simulink model "drone_nonlinear_full_identification2"  (R2018a)
settings: Solver=VariableStepAuto  StartTime=0.0  StopTime=40  RelTol=1e-3
undefined symbols (not defined in the file): g, Ix, Iy, Iz, m, simulation_sampling_ts
libraries: simulink x4
settings Model: Creator=ros  LastModifiedBy=ros

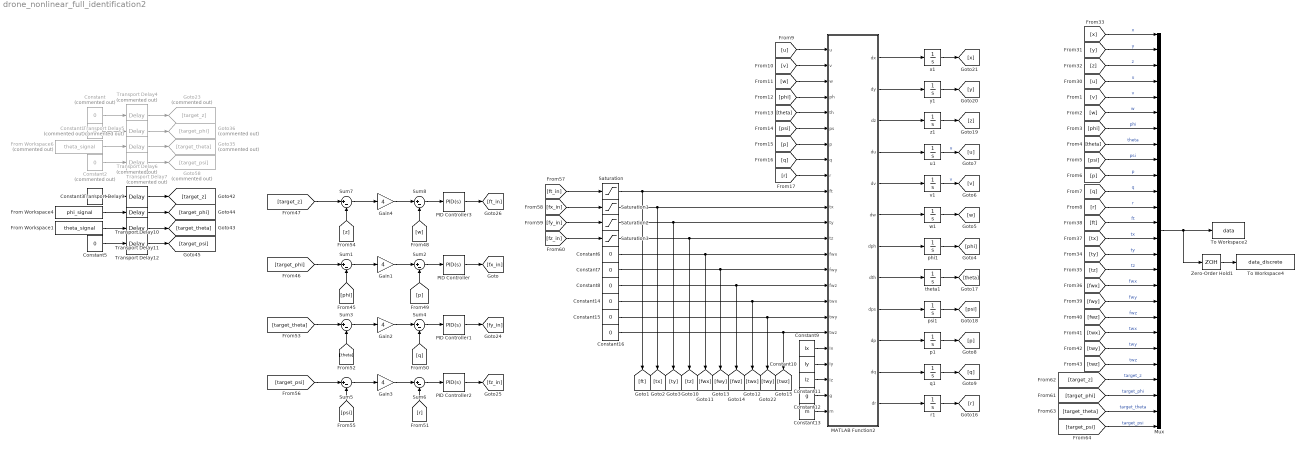
== system drone_nonlinear_full_identification2 ==
  Constant : Constant  Commented=on  Value=0
  Constant1 : Constant  Commented=on  Value=0
  Constant10 : Constant  Value=Iy
  Constant11 : Constant  Value=Iz
  Constant12 : Constant  Value=g
  Constant13 : Constant  Value=m
  Constant{3,5..8,14..16} (8 alike) : Constant  Value=0
  Constant2 : Constant  Commented=on  Value=0
  Constant9 : Constant  Value=Ix
  From Workspace1 : FromWorkspace  VariableName=theta_signal  SampleTime=0
  From Workspace4 : FromWorkspace  VariableName=phi_signal  SampleTime=0
  From Workspace6 : FromWorkspace  Commented=on  VariableName=theta_signal  SampleTime=0
  Gain{1..4} (4 alike) : Gain  Gain=4
  Goto23 : Goto  Commented=on  GotoTag=target_z
  Goto35 : Goto  Commented=on  GotoTag=target_theta
  Goto36 : Goto  Commented=on  GotoTag=target_phi
  Goto58 : Goto  Commented=on  GotoTag=target_psi
  MATLAB Function2 : MATLAB Function  TreatAsAtomicUnit=on
  Mux : Mux  Inputs=26
  PID Controller : simulink/Continuous/PID Controller  Controller=PID  TimeDomain=Continuous-time  SampleTime=-1  IntegratorMethod=Forward Euler  FilterMethod=Forward Euler  Form=Parallel  UseFilter=on  ControllerParametersSource=internal  P=1.5  I=1.5  D=0  N=100  InitialConditionSource=internal  InitialConditionForIntegrator=0  InitialConditionForFilter=0  ExternalReset=none  LimitOutput=off  UpperSaturationLimit=inf  LowerSaturationLimit=-inf  LinearizeAsGain=on  AntiWindupMode=none  Kb=1  TrackingMode=off  Kt=1  PParamMin=[]  PParamMax=[]  IParamMin=[]  IParamMax=[]  DParamMin=[]  DParamMax=[]  NParamMin=[]  NParamMax=[]  KbParamMin=[]  KbParamMax=[]  KtParamMin=[]  KtParamMax=[]  POutMin=[]  POutMax=[]  IOutMin=[]  IOutMax=[]  DOutMin=[]  DOutMax=[]  NOutMin=[]  NOutMax=[]  KbOutMin=[]  KbOutMax=[]  KtOutMin=[]  KtOutMax=[]  IntegratorOutMin=[]  IntegratorOutMax=[]  FilterOutMin=[]  FilterOutMax=[]  SumOutMin=[]  SumOutMax=[]  SumI1OutMin=[]  SumI1OutMax=[]  SumI2OutMin=[]  SumI2OutMax=[]  SumI3OutMin=[]  SumI3OutMax=[]  SumDOutMin=[]  SumDOutMax=[]  SaturationOutMin=[]  SaturationOutMax=[]  IntegratorContinuousStateAttributes=''  IntegratorStateMustResolveToSignalObject=off  IntegratorRTWStateStorageClass=Auto  FilterContinuousStateAttributes=''  FilterStateMustResolveToSignalObject=off  FilterRTWStateStorageClass=Auto  DifferentiatorICPrevScaledInput=0  DifferentiatorOutMin=[]  DifferentiatorOutMax=[]  FilterDiffOutCoefMin=[]  FilterDiffOutCoefMax=[]  SumDenOutMin=[]  SumDenOutMax=[]  SumNumOutMin=[]  SumNumOutMax=[]  ReciprocalOutMin=[]  ReciprocalOutMax=[]  DivideOutMin=[]  DivideOutMax=[]  TunerSelectOption=Transfer Function Based (PID Tuner App)
  PID Controller1 : simulink/Continuous/PID Controller  Controller=PID  TimeDomain=Continuous-time  SampleTime=-1  IntegratorMethod=Forward Euler  FilterMethod=Forward Euler  Form=Parallel  UseFilter=on  ControllerParametersSource=internal  P=1.5  I=1.5  D=0  N=100  InitialConditionSource=internal  InitialConditionForIntegrator=0  InitialConditionForFilter=0  ExternalReset=none  LimitOutput=off  UpperSaturationLimit=inf  LowerSaturationLimit=-inf  LinearizeAsGain=on  AntiWindupMode=none  Kb=1  TrackingMode=off  Kt=1  PParamMin=[]  PParamMax=[]  IParamMin=[]  IParamMax=[]  DParamMin=[]  DParamMax=[]  NParamMin=[]  NParamMax=[]  KbParamMin=[]  KbParamMax=[]  KtParamMin=[]  KtParamMax=[]  POutMin=[]  POutMax=[]  IOutMin=[]  IOutMax=[]  DOutMin=[]  DOutMax=[]  NOutMin=[]  NOutMax=[]  KbOutMin=[]  KbOutMax=[]  KtOutMin=[]  KtOutMax=[]  IntegratorOutMin=[]  IntegratorOutMax=[]  FilterOutMin=[]  FilterOutMax=[]  SumOutMin=[]  SumOutMax=[]  SumI1OutMin=[]  SumI1OutMax=[]  SumI2OutMin=[]  SumI2OutMax=[]  SumI3OutMin=[]  SumI3OutMax=[]  SumDOutMin=[]  SumDOutMax=[]  SaturationOutMin=[]  SaturationOutMax=[]  IntegratorContinuousStateAttributes=''  IntegratorStateMustResolveToSignalObject=off  IntegratorRTWStateStorageClass=Auto  FilterContinuousStateAttributes=''  FilterStateMustResolveToSignalObject=off  FilterRTWStateStorageClass=Auto  DifferentiatorICPrevScaledInput=0  DifferentiatorOutMin=[]  DifferentiatorOutMax=[]  FilterDiffOutCoefMin=[]  FilterDiffOutCoefMax=[]  SumDenOutMin=[]  SumDenOutMax=[]  SumNumOutMin=[]  SumNumOutMax=[]  ReciprocalOutMin=[]  ReciprocalOutMax=[]  DivideOutMin=[]  DivideOutMax=[]  TunerSelectOption=Transfer Function Based (PID Tuner App)
  PID Controller2 : simulink/Continuous/PID Controller  Controller=PID  TimeDomain=Continuous-time  SampleTime=-1  IntegratorMethod=Forward Euler  FilterMethod=Forward Euler  Form=Parallel  UseFilter=on  ControllerParametersSource=internal  P=1.5  I=1.5  D=0  N=100  InitialConditionSource=internal  InitialConditionForIntegrator=0  InitialConditionForFilter=0  ExternalReset=none  LimitOutput=off  UpperSaturationLimit=inf  LowerSaturationLimit=-inf  LinearizeAsGain=on  AntiWindupMode=none  Kb=1  TrackingMode=off  Kt=1  PParamMin=[]  PParamMax=[]  IParamMin=[]  IParamMax=[]  DParamMin=[]  DParamMax=[]  NParamMin=[]  NParamMax=[]  KbParamMin=[]  KbParamMax=[]  KtParamMin=[]  KtParamMax=[]  POutMin=[]  POutMax=[]  IOutMin=[]  IOutMax=[]  DOutMin=[]  DOutMax=[]  NOutMin=[]  NOutMax=[]  KbOutMin=[]  KbOutMax=[]  KtOutMin=[]  KtOutMax=[]  IntegratorOutMin=[]  IntegratorOutMax=[]  FilterOutMin=[]  FilterOutMax=[]  SumOutMin=[]  SumOutMax=[]  SumI1OutMin=[]  SumI1OutMax=[]  SumI2OutMin=[]  SumI2OutMax=[]  SumI3OutMin=[]  SumI3OutMax=[]  SumDOutMin=[]  SumDOutMax=[]  SaturationOutMin=[]  SaturationOutMax=[]  IntegratorContinuousStateAttributes=''  IntegratorStateMustResolveToSignalObject=off  IntegratorRTWStateStorageClass=Auto  FilterContinuousStateAttributes=''  FilterStateMustResolveToSignalObject=off  FilterRTWStateStorageClass=Auto  DifferentiatorICPrevScaledInput=0  DifferentiatorOutMin=[]  DifferentiatorOutMax=[]  FilterDiffOutCoefMin=[]  FilterDiffOutCoefMax=[]  SumDenOutMin=[]  SumDenOutMax=[]  SumNumOutMin=[]  SumNumOutMax=[]  ReciprocalOutMin=[]  ReciprocalOutMax=[]  DivideOutMin=[]  DivideOutMax=[]  TunerSelectOption=Transfer Function Based (PID Tuner App)
  PID Controller3 : simulink/Continuous/PID Controller  Controller=PID  TimeDomain=Continuous-time  SampleTime=-1  IntegratorMethod=Forward Euler  FilterMethod=Forward Euler  Form=Parallel  UseFilter=on  ControllerParametersSource=internal  P=7  I=6  D=0.7  N=100  InitialConditionSource=internal  InitialConditionForIntegrator=0  InitialConditionForFilter=0  ExternalReset=none  LimitOutput=off  UpperSaturationLimit=inf  LowerSaturationLimit=-inf  LinearizeAsGain=on  AntiWindupMode=none  Kb=1  TrackingMode=off  Kt=1  PParamMin=[]  PParamMax=[]  IParamMin=[]  IParamMax=[]  DParamMin=[]  DParamMax=[]  NParamMin=[]  NParamMax=[]  KbParamMin=[]  KbParamMax=[]  KtParamMin=[]  KtParamMax=[]  POutMin=[]  POutMax=[]  IOutMin=[]  IOutMax=[]  DOutMin=[]  DOutMax=[]  NOutMin=[]  NOutMax=[]  KbOutMin=[]  KbOutMax=[]  KtOutMin=[]  KtOutMax=[]  IntegratorOutMin=[]  IntegratorOutMax=[]  FilterOutMin=[]  FilterOutMax=[]  SumOutMin=[]  SumOutMax=[]  SumI1OutMin=[]  SumI1OutMax=[]  SumI2OutMin=[]  SumI2OutMax=[]  SumI3OutMin=[]  SumI3OutMax=[]  SumDOutMin=[]  SumDOutMax=[]  SaturationOutMin=[]  SaturationOutMax=[]  IntegratorContinuousStateAttributes=''  IntegratorStateMustResolveToSignalObject=off  IntegratorRTWStateStorageClass=Auto  FilterContinuousStateAttributes=''  FilterStateMustResolveToSignalObject=off  FilterRTWStateStorageClass=Auto  DifferentiatorICPrevScaledInput=0  DifferentiatorOutMin=[]  DifferentiatorOutMax=[]  FilterDiffOutCoefMin=[]  FilterDiffOutCoefMax=[]  SumDenOutMin=[]  SumDenOutMax=[]  SumNumOutMin=[]  SumNumOutMax=[]  ReciprocalOutMin=[]  ReciprocalOutMax=[]  DivideOutMin=[]  DivideOutMax=[]  TunerSelectOption=Transfer Function Based (PID Tuner App)
  Saturation{,1..3} (4 alike) : Saturate  UpperLimit=30  LowerLimit=-100
  Sum{1..8} (8 alike) : Sum  Inputs=|+-
  To Workspace2 : ToWorkspace  VariableName=data  SaveFormat=Timeseries  SampleTime=-1
  To Workspace4 : ToWorkspace  VariableName=data_discrete  SaveFormat=Timeseries  SampleTime=-1
  Transport Delay{9..12} (4 alike) : TransportDelay  DelayTime=10
  Transport Delay{4..7} (4 alike) : TransportDelay  Commented=on  DelayTime=10
  Zero-Order Hold1 : ZeroOrderHold  SampleTime=simulation_sampling_ts
  p1 : Integrator
  phi1 : Integrator
  psi1 : Integrator
  q1 : Integrator
  r1 : Integrator
  theta1 : Integrator
  u1 : Integrator
  v1 : Integrator
  w1 : Integrator
  x1 : Integrator
  y1 : Integrator
  z1 : Integrator
  wires:
  [v] -> MATLAB Function2/2(v)
  MATLAB Function2/9(dps) -> psi1/1
  MATLAB Function2/10(dp) -> p1/1
  MATLAB Function2/5(dv) -> v1/1
  [r] -> MATLAB Function2/9(r)
  [psi] -> MATLAB Function2/6(ps)
  [p] -> MATLAB Function2/7(p)
  p1/1 -> [p]
  MATLAB Function2/12(dr) -> r1/1
  theta1/1 -> [theta]
  [w] -> MATLAB Function2/3(w)
  [phi] -> MATLAB Function2/4(ph)
  [q] -> MATLAB Function2/8(q)
  r1/1 -> [r]
  q1/1 -> [q]
  MATLAB Function2/11(dq) -> q1/1
  MATLAB Function2/6(dw) -> w1/1
  MATLAB Function2/4(du) -> u1/1
  psi1/1 -> [psi]
  [u] -> MATLAB Function2/1(u)
  MATLAB Function2/8(dth) -> theta1/1
  [theta] -> MATLAB Function2/5(th)
  u1/1 -> [u]  "u"
  w1/1 -> [w]
  MATLAB Function2/7(dph) -> phi1/1
  v1/1 -> [v]  "v"
  Constant9/1 -> MATLAB Function2/20(Ix)
  Constant13/1 -> MATLAB Function2/24(m)
  Constant11/1 -> MATLAB Function2/22(Iz)
  Constant10/1 -> MATLAB Function2/21(Iy)
  Constant12/1 -> MATLAB Function2/23(g)
  MATLAB Function2/1(dx) -> x1/1
  MATLAB Function2/2(dy) -> y1/1
  MATLAB Function2/3(dz) -> z1/1
  Constant6/1 -> [fwx], MATLAB Function2/14(fwx)
  Constant7/1 -> [fwy], MATLAB Function2/15(fwy)
  Constant14/1 -> [twx], MATLAB Function2/17(twx)
  Constant8/1 -> [fwz], MATLAB Function2/16(fwz)
  Constant15/1 -> [twy], MATLAB Function2/18(twy)
  Constant16/1 -> [twz], MATLAB Function2/19(twz)
  z1/1 -> [z]
  y1/1 -> [y]
  x1/1 -> [x]
  [x] -> Mux/1  "x"
  [v] -> Mux/5  "v"
  [z] -> Mux/3  "z"
  [w] -> Mux/6  "w"
  [p] -> Mux/10  "p"
  [phi] -> Mux/7  "phi"
  [theta] -> Mux/8  "theta"
  [r] -> Mux/12  "r"
  [y] -> Mux/2  "y"
  [psi] -> Mux/9  "psi"
  [u] -> Mux/4  "u"
  [q] -> Mux/11  "q"
  Mux/1 -> Zero-Order Hold1/1, To Workspace2/1
  [ft] -> Mux/13  "ft"
  [tx] -> Mux/14  "tx"
  [ty] -> Mux/15  "ty"
  [tz] -> Mux/16  "tz"
  [fwx] -> Mux/17  "fwx"
  [fwy] -> Mux/18  "fwy"
  [fwz] -> Mux/19  "fwz"
  [twx] -> Mux/20  "twx"
  [twy] -> Mux/21  "twy"
  [twz] -> Mux/22  "twz"
  phi1/1 -> [phi]
  Zero-Order Hold1/1 -> To Workspace4/1
  [phi] -> Sum1/2
  [target_phi] -> Sum1/1
  Sum1/1 -> Gain1/1
  Gain1/1 -> Sum2/1
  Sum2/1 -> PID Controller/1
  [p] -> Sum2/2
  [q] -> Sum4/2
  Gain2/1 -> Sum4/1
  [target_theta] -> Sum3/1
  Sum4/1 -> PID Controller1/1
  Sum3/1 -> Gain2/1
  [theta] -> Sum3/2
  [r] -> Sum6/2
  Gain3/1 -> Sum6/1
  [target_psi] -> Sum5/1
  Sum6/1 -> PID Controller2/1
  Sum5/1 -> Gain3/1
  [psi] -> Sum5/2
  [target_z] -> Sum7/1
  Sum8/1 -> PID Controller3/1
  [w] -> Sum8/2
  Sum7/1 -> Gain4/1
  Gain4/1 -> Sum8/1
  [z] -> Sum7/2
  PID Controller/1 -> [fx_in]
  PID Controller2/1 -> [fz_in]
  PID Controller1/1 -> [fy_in]
  PID Controller3/1 -> [ft_in]
  Saturation/1 -> [ft], MATLAB Function2/10(ft)
  Saturation1/1 -> [tx], MATLAB Function2/11(tx)
  Saturation2/1 -> [ty], MATLAB Function2/12(ty)
  Saturation3/1 -> [tz], MATLAB Function2/13(tz)
  [target_z] -> Mux/23  "target_z"
  [target_phi] -> Mux/24  "target_phi"
  [target_theta] -> Mux/25  "target_theta"
  [target_psi] -> Mux/26  "target_psi"
  [ft_in] -> Saturation/1
  [fx_in] -> Saturation1/1
  [fy_in] -> Saturation2/1
  [fz_in] -> Saturation3/1
  Transport Delay10/1 -> [target_phi]
  Transport Delay9/1 -> [target_z]
  Transport Delay12/1 -> [target_psi]
  From Workspace1/1 -> Transport Delay11/1
  Constant3/1 -> Transport Delay9/1
  Transport Delay7/1 -> Goto58/1
  From Workspace4/1 -> Transport Delay10/1
  Transport Delay11/1 -> [target_theta]
  Constant/1 -> Transport Delay4/1
  Constant5/1 -> Transport Delay12/1
  Constant2/1 -> Transport Delay7/1
  Constant1/1 -> Transport Delay5/1
  Transport Delay4/1 -> Goto23/1
  From Workspace6/1 -> Transport Delay6/1
  Transport Delay6/1 -> Goto35/1
  Transport Delay5/1 -> Goto36/1

== matlab function drone_nonlinear_full_identification2/MATLAB Function2 ==
  data: u input; v input; dx output; w input; ph input; th input; ps input; p input; q input; r input; ft input; tx input; ty input; tz input; fwx input; fwy input; fwz input; twx input; twy input; twz input; dy output; dz output; du output; dv output; dw output; dph output; dth output; dps output; dp output; dq output; dr output; Ix input; Iy input; Iz input; g input; m input
function [dx, dy, dz, du, dv, dw, dph, dth, dps, dp, dq, dr] = fcn(u, v, w, ph, th, ps, p, q, r, ft, tx, ty, tz, fwx, fwy, fwz, twx, twy, twz, Ix, Iy, Iz, g, m)

dx = w*(sin(ph)*sin(ps) + cos(ph)*cos(ps)*sin(th)) - v*(cos(ph)*sin(ps) - cos(ps)*sin(ph)*sin(th)) + u*(cos(ps)*cos(th));
dy = v*(cos(ph)*cos(ps) + sin(ph)*sin(ps)*sin(th)) - w*(cos(ps)*sin(ph) - cos(ph)*sin(ps)*sin(th)) + u*(cos(th)*sin(ps));
dz = w*(cos(ph)*cos(th)) - u*(sin(th)) + v*(cos(th)*sin(ph));
du = r*v - q*w + g*(sin(th)) + fwx / m;
dv = p*w - r*u - g*(sin(ph)*cos(th)) + fwy / m;
dw = q*u - p*v - g*(cos(th)*cos(ph)) + (fwz + ft) / m;
dph = p + r*(cos(ph)*tan(th)) + q*(sin(ph)*tan(th));
dth = q*(cos(th)) - r*(sin(ph));
dps = r*(cos(ph)/cos(th)) + q*(sin(ph)/cos(th));
dp = r*q*(Iy - Iz)/Ix + (tx + twx)/Ix;
dq = p*r*(Iz - Ix)/Iy + (ty + twy)/Iy;
dr = p*q*(Ix - Iy)/Iz + (tz + twz)/Iz;
